simulink model "controladorBorroso"  (R2019a)
settings: Solver=VariableStepAuto  StartTime=0.0  StopTime=10.0  RelTol=1e-3
libraries: fuzblock x1
settings Model: Creator=Alumno  LastModifiedBy=Alumno

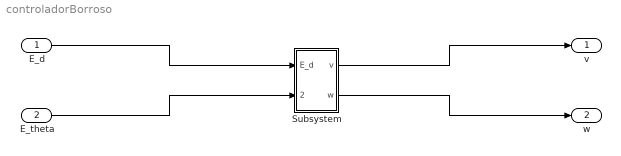
== system controladorBorroso ==
  "E_d " : Inport
  E_theta : Inport  Port=2
  Subsystem : Subsystem
  v : Outport
  w : Outport  Port=2
  wires:
  "E_d "/1 -> Subsystem/1("E_d ")
  E_theta/1 -> Subsystem/2(E_theta)
  Subsystem/1(v) -> v/1
  Subsystem/2(w) -> w/1

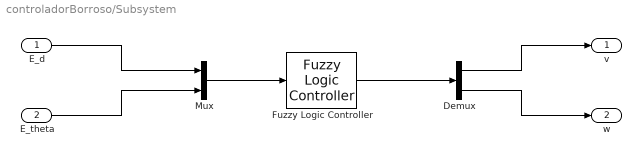
== system controladorBorroso/Subsystem ==
  "E_d " : Inport
  E_theta : Inport  Port=2
  Demux : Demux  Outputs=2
  Fuzzy Logic Controller : fuzblock/Fuzzy Logic  Controller  FIS='practica2.fis'  OutputSampleNumber=101  DataType=double  FuzzifiedInputs=off  RuleFiringStrengths=off  RuleOutputs=off  AggregatedOutputs=off  SimulateUsing=Interpreted execution  OutOfRangeInputValueMessage=warning  NoRuleFiredMessage=warning  EmptyOutputFuzzySetMessage=warning
  Mux : Mux  Inputs=2
  v : Outport
  w : Outport  Port=2
  wires:
  Mux/1 -> Fuzzy Logic Controller/1
  Demux/1 -> v/1
  "E_d "/1 -> Mux/1
  E_theta/1 -> Mux/2
  Demux/2 -> w/1
  Fuzzy Logic Controller/1 -> Demux/1
